simulink model "testPID_RollRotation"  (R2021a)
settings: Solver=VariableStepAuto  StartTime=0.0  StopTime=Torb  RelTol=1e-3
libraries: simulink x1, sharedtransform x1
settings Model: DataDictionary=databus.sldd  Creator=Laura  LastModifiedBy=Laura

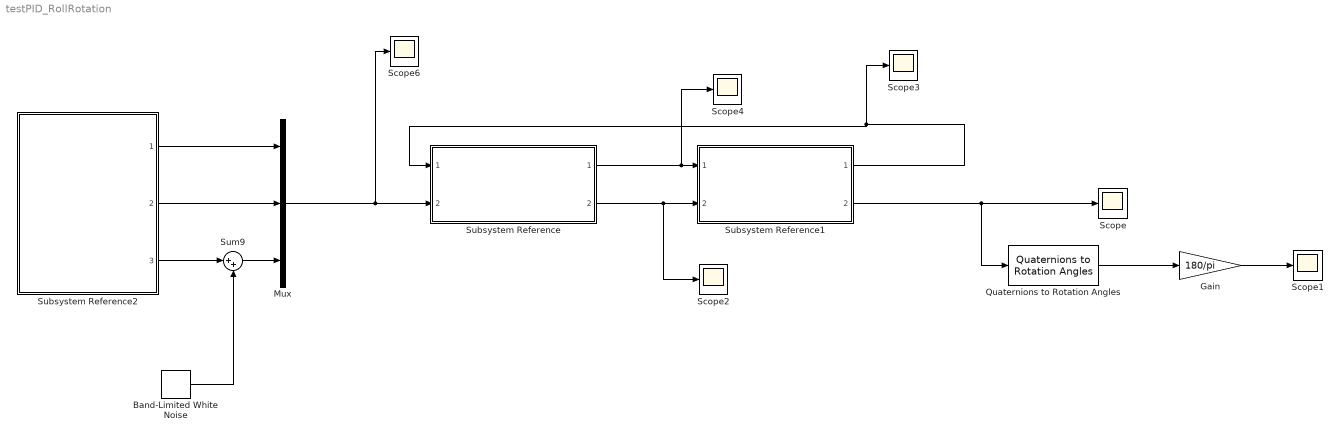
== system testPID_RollRotation ==
  Band-Limited White Noise : simulink/Sources/Band-Limited White Noise  Cov=[1e-11]  Ts=0.1  seed=[23341]
  Gain : Gain  Gain=180/pi
  Mux : Mux  Inputs=3
  Quaternions to Rotation Angles : sharedtransform/Quaternions to Rotation Angles  rotationOrder=ZYX  aMode=aMode
      settings: SourceProductBaseCode=AE,PW,DR,MT,UV,VE
  Scope{,1..4,6} (6 alike) : Scope
  Subsystem Reference : Subsystem  ReferencedSubsystem=Dynamics
  Subsystem Reference1 : Subsystem  ReferencedSubsystem=Kinematics
  Subsystem Reference2 : Subsystem  ReferencedSubsystem=ThrustSignals
  Sum9 : Sum  Inputs=|++
  wires:
  Subsystem Reference1/1 -> Scope3/1, Subsystem Reference/1
  Subsystem Reference1/2 -> Quaternions to Rotation Angles/1, Scope/1
  Subsystem Reference/2 -> Scope2/1, Subsystem Reference1/2
  Subsystem Reference/1 -> Scope4/1, Subsystem Reference1/1
  Quaternions to Rotation Angles/1 -> Gain/1
  Gain/1 -> Scope1/1
  Subsystem Reference2/1 -> Mux/1
  Mux/1 -> Subsystem Reference/2, Scope6/1
  Subsystem Reference2/2 -> Mux/2
  Sum9/1 -> Mux/3
  Subsystem Reference2/3 -> Sum9/1
  Band-Limited White Noise/1 -> Sum9/2
